simulink model "distance_kf_sim"  (R2017a)
settings: Solver=VariableStepAuto  StartTime=0.0  StopTime=10.0  RelTol=1e-3
settings Model: Creator=cg  LastModifiedBy=cg

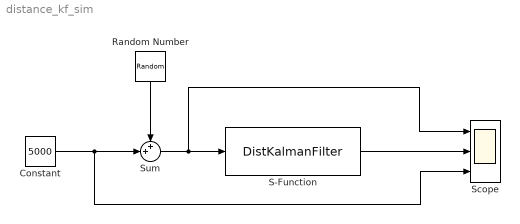
== system distance_kf_sim ==
  Constant : Constant  Value=5000
  Random Number : RandomNumber  Variance=5  SampleTime=0.1
  S-Function : S-Function  FunctionName=DistKalmanFilter  SFunctionDeploymentMode=off  EnableBusSupport=off
  Scope : Scope  NumInputPorts=3
  Sum : Sum  Inputs=++|
  wires:
  Sum/1 -> Scope/1, S-Function/1
  S-Function/1 -> Scope/2
  Random Number/1 -> Sum/1
  Constant/1 -> Scope/3, Sum/2
